simulink model "exp_07_a"  (R2018b)
settings: Solver=VariableStepAuto  StartTime=0.0  StopTime=10.0  RelTol=1e-3
settings Model: Creator=student  LastModifiedBy=student

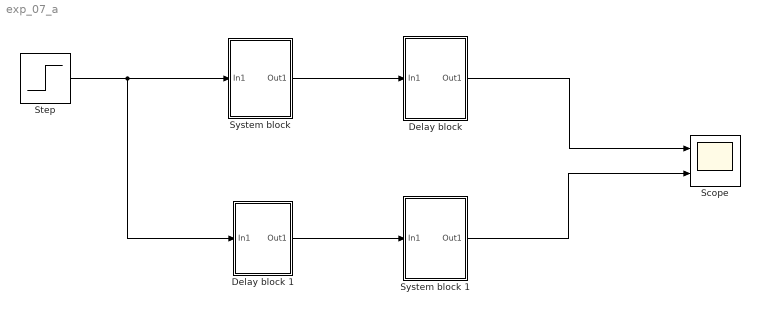
== system exp_07_a ==
  Delay block : Subsystem
  Delay block 1 : Subsystem
  Scope : Scope  NumInputPorts=2
  Step : Step  SampleTime=0
  System block : Subsystem
  System block 1 : Subsystem
  wires:
  Step/1 -> System block/1(In1), Delay block 1/1(In1)
  System block/1(Out1) -> Delay block/1(In1)
  Delay block/1(Out1) -> Scope/1
  Delay block 1/1(Out1) -> System block 1/1(In1)
  System block 1/1(Out1) -> Scope/2

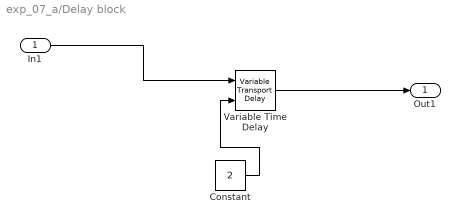
== system exp_07_a/Delay block ==
  In1 : Inport
  Constant : Constant  Value=2
  Variable Time Delay : VariableTransportDelay  MaximumDelay=10
  Out1 : Outport
  wires:
  Variable Time Delay/1 -> Out1/1
  Constant/1 -> Variable Time Delay/2
  In1/1 -> Variable Time Delay/1

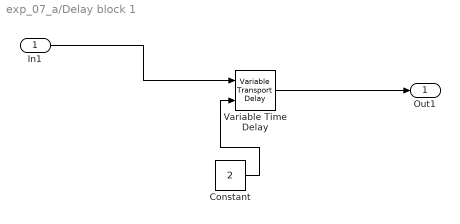
== system exp_07_a/Delay block 1 ==
  In1 : Inport
  Constant : Constant  Value=2
  Variable Time Delay : VariableTransportDelay  MaximumDelay=10
  Out1 : Outport
  wires:
  Variable Time Delay/1 -> Out1/1
  Constant/1 -> Variable Time Delay/2
  In1/1 -> Variable Time Delay/1

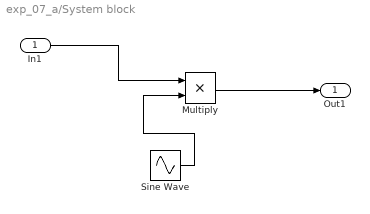
== system exp_07_a/System block ==
  In1 : Inport
  Multiply : Product
  Sine Wave : Sin  SampleTime=0
  Out1 : Outport
  wires:
  Sine Wave/1 -> Multiply/2
  In1/1 -> Multiply/1
  Multiply/1 -> Out1/1

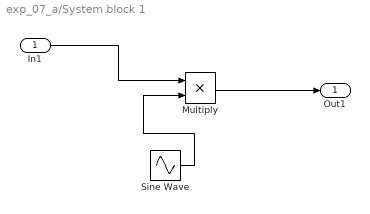
== system exp_07_a/System block 1 ==
  In1 : Inport
  Multiply : Product
  Sine Wave : Sin  SampleTime=0
  Out1 : Outport
  wires:
  Sine Wave/1 -> Multiply/2
  In1/1 -> Multiply/1
  Multiply/1 -> Out1/1
